simulink model "model"  (R2018b)
settings: Solver=ode4  StartTime=0.0  StopTime=10  FixedStep=0.005  RelTol=1e-3  EnableMultiTasking=on
settings Model: Creator=Administrator  LastModifiedBy=q5461
settings DataIOCC: LimitDataPoints=on
settings OptimizationCC: LifeSpan=inf
settings DebuggingCC: AllowSymbolicDim=off  SFUnexpectedBacktrackingDiag=warning  SFNoUnconditionalDefaultTransitionDiag=warning  SFExecutionAtInitializationDiag=none
settings ModelReferenceCC: PropagateSignalLabelsOutOfModel=off
settings SFSimCC: SimUseLocalCustomCode=off
settings RTWCC: RTWUseLocalCustomCode=off
settings CodeAppCC: StateflowObjectComments=on
settings GRTTargetCC: TargetLangStandard=C89/C90 (ANSI)
settings ConfigComp: CovMetricSettings=dw  CovHtmlReporting=on  CovSaveCumulativeToWorkspaceVar=on  CovSaveSingleToWorkspaceVar=on  CovExternalEMLEnable=off

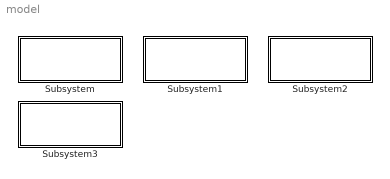
== system model ==
  Subsystem : Subsystem
  Subsystem1 : Subsystem
  Subsystem2 : Subsystem
  Subsystem3 : Subsystem

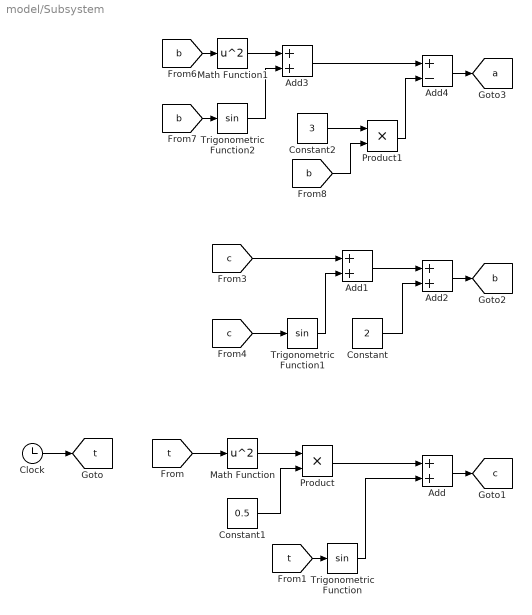
== system model/Subsystem ==
  Add{,1..3} (4 alike) : Sum
  Add4 : Sum  Inputs=+-
  Clock : Clock
  Constant : Constant  Value=2
  Constant1 : Constant  Value=0.5
  Constant2 : Constant  Value=3
  Math Function : Math  Operator=square  SaturateOnIntegerOverflow=on
  Math Function1 : Math  Operator=square  SaturateOnIntegerOverflow=on
  Product : Product
  Product1 : Product
  Trigonometric Function : Trigonometry
  Trigonometric Function1 : Trigonometry
  Trigonometric Function2 : Trigonometry
  tag scope: a=global, b=global, c=global, t=global
  wires:
  Math Function1/1 -> Add3/1
  Clock/1 -> [t]
  [b] -> Trigonometric Function2/1
  Add4/1 -> [a]
  [b] -> Product1/2
  Add3/1 -> Add4/1
  Constant2/1 -> Product1/1
  [b] -> Math Function1/1
  Add/1 -> [c]
  Trigonometric Function2/1 -> Add3/2
  [c] -> Add1/1
  Add1/1 -> Add2/1
  Trigonometric Function/1 -> Add/2
  Add2/1 -> [b]
  Trigonometric Function1/1 -> Add1/2
  Constant/1 -> Add2/2
  [t] -> Trigonometric Function/1
  [t] -> Math Function/1
  Constant1/1 -> Product/2
  Product/1 -> Add/1
  Product1/1 -> Add4/2
  Math Function/1 -> Product/1
  [c] -> Trigonometric Function1/1

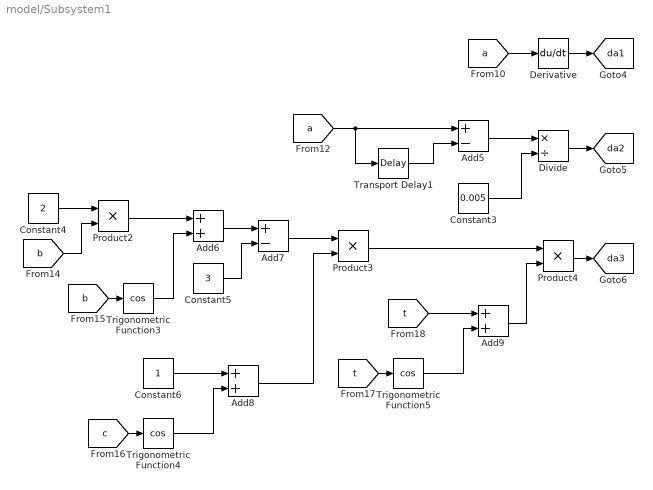
== system model/Subsystem1 ==
  Add5 : Sum  Inputs=+-
  Add6 : Sum
  Add7 : Sum  Inputs=+-
  Add8 : Sum
  Add9 : Sum
  Constant3 : Constant  Value=0.005
  Constant4 : Constant  Value=2
  Constant5 : Constant  Value=3
  Constant6 : Constant
  Derivative : Derivative
  Divide : Product  Inputs=*/
  Product2 : Product
  Product3 : Product
  Product4 : Product
  Transport Delay1 : TransportDelay  DelayTime=0.005
  Trigonometric Function3 : Trigonometry  Operator=cos
  Trigonometric Function4 : Trigonometry  Operator=cos
  Trigonometric Function5 : Trigonometry  Operator=cos
  tag scope: da1=global, da2=global, da3=global
  wires:
  Constant5/1 -> Add7/2
  [b] -> Product2/2
  Derivative/1 -> [da1]
  [a] -> Transport Delay1/1, Add5/1
  [b] -> Trigonometric Function3/1
  Add9/1 -> Product4/2
  Trigonometric Function5/1 -> Add9/2
  [t] -> Add9/1
  Trigonometric Function3/1 -> Add6/2
  Constant6/1 -> Add8/1
  Add6/1 -> Add7/1
  Add8/1 -> Product3/2
  Constant4/1 -> Product2/1
  Transport Delay1/1 -> Add5/2
  Product2/1 -> Add6/1
  Add5/1 -> Divide/1
  Product4/1 -> [da3]
  Constant3/1 -> Divide/2
  [t] -> Trigonometric Function5/1
  Divide/1 -> [da2]
  Add7/1 -> Product3/1
  Trigonometric Function4/1 -> Add8/2
  [a] -> Derivative/1
  [c] -> Trigonometric Function4/1
  Product3/1 -> Product4/1

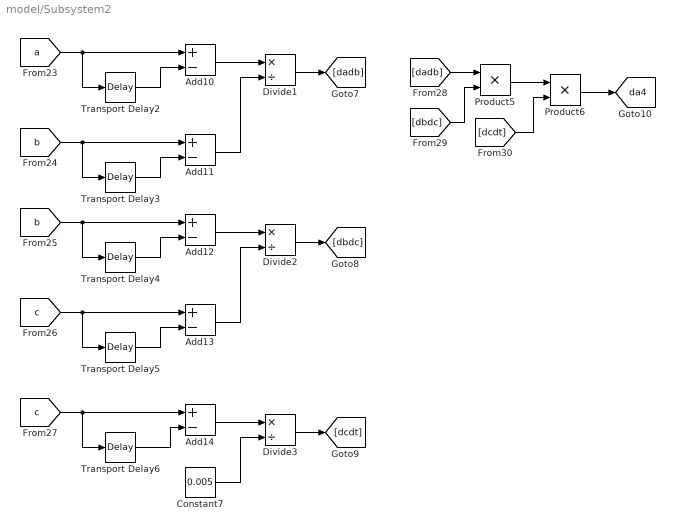
== system model/Subsystem2 ==
  Add{10..14} (5 alike) : Sum  Inputs=+-
  Constant7 : Constant  Value=0.005
  Divide1 : Product  Inputs=*/
  Divide2 : Product  Inputs=*/
  Divide3 : Product  Inputs=*/
  Product5 : Product
  Product6 : Product
  Transport Delay{2..6} (5 alike) : TransportDelay  DelayTime=0.005
  tag scope: da4=global
  wires:
  Add14/1 -> Divide3/1
  Divide2/1 -> [dbdc]
  Add11/1 -> Divide1/2
  [dadb] -> Product5/1
  Product5/1 -> Product6/1
  Transport Delay5/1 -> Add13/2
  Transport Delay4/1 -> Add12/2
  Add12/1 -> Divide2/1
  Transport Delay3/1 -> Add11/2
  Constant7/1 -> Divide3/2
  [c] -> Transport Delay6/1, Add14/1
  [b] -> Transport Delay3/1, Add11/1
  Transport Delay6/1 -> Add14/2
  [b] -> Transport Delay4/1, Add12/1
  [dbdc] -> Product5/2
  Transport Delay2/1 -> Add10/2
  [dcdt] -> Product6/2
  Add10/1 -> Divide1/1
  [a] -> Add10/1, Transport Delay2/1
  [c] -> Add13/1, Transport Delay5/1
  Divide1/1 -> [dadb]
  Product6/1 -> [da4]
  Add13/1 -> Divide2/2
  Divide3/1 -> [dcdt]

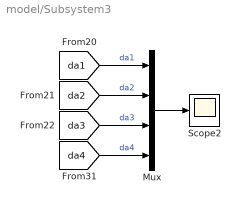
== system model/Subsystem3 ==
  Mux : Mux
  Scope2 : Scope
  wires:
  Mux/1 -> Scope2/1
  [da3] -> Mux/3  "da3"
  [da2] -> Mux/2  "da2"
  [da4] -> Mux/4  "da4"
  [da1] -> Mux/1  "da1"
